simulink model "ClassicalController"  (R2021a)
settings: Solver=VariableStepAuto  StartTime=0.0  StopTime=200  RelTol=1e-3
values from neighbouring files (symbols this model uses):
  Sim_A = m.EquilibriumStateSpace.A    [main.m]
  Sim_B = m.EquilibriumStateSpace.B    [main.m]
  Sim_C = m.EquilibriumStateSpace.C    [main.m]
  Sim_c1_d = sym2poly(d)    [main.m]
  Sim_c1_n = sym2poly(n)    [main.m]
  Sim_c2_d = sym2poly(d)    [main.m]
  Sim_c2_n = sym2poly(n)    [main.m]
settings Model: Creator=james  LastModifiedBy=james

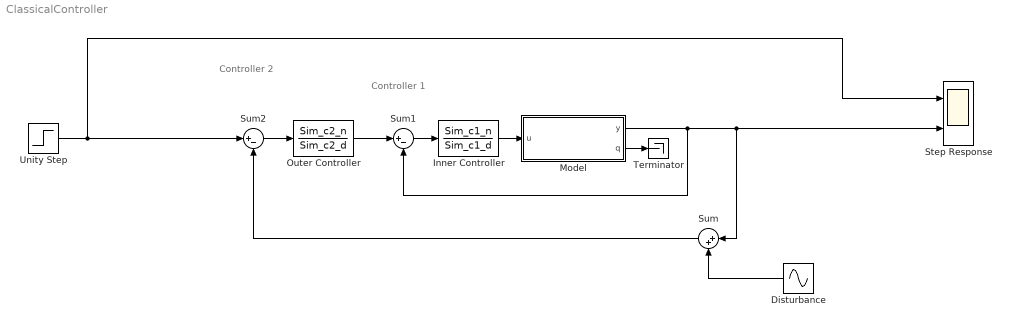
== system ClassicalController ==
  note: Controller 2
  note: Controller 1
  Disturbance : Sin  Amplitude=0.5  Frequency=50  SampleTime=0
  Inner Controller : TransferFcn  Numerator=Sim_c1_n  Denominator=Sim_c1_d
  Model : Subsystem
  Outer Controller : TransferFcn  Numerator=Sim_c2_n  Denominator=Sim_c2_d
  Step Response : Scope  NumInputPorts=2
  Sum : Sum  Inputs=|++
  Sum1 : Sum  Inputs=|+-
  Sum2 : Sum  Inputs=|+-
  Terminator : Terminator
  Unity Step : Step  SampleTime=0
  wires:
  Model/1(y) -> Sum1/2, Sum/1, Step Response/2
  Sum1/1 -> Inner Controller/1
  Model/2(q) -> Terminator/1
  Inner Controller/1 -> Model/1(u)
  Outer Controller/1 -> Sum1/1
  Sum2/1 -> Outer Controller/1
  Unity Step/1 -> Sum2/1, Step Response/1
  Sum/1 -> Sum2/2
  Disturbance/1 -> Sum/2

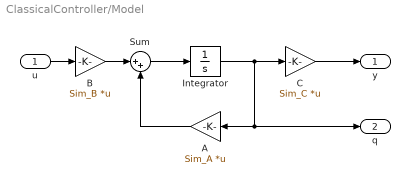
== system ClassicalController/Model ==
  u : Inport
  A : Gain  Gain=Sim_A  Multiplication=Matrix(K*u)
  B : Gain  Gain=Sim_B  Multiplication=Matrix(K*u)
  C : Gain  Gain=Sim_C  Multiplication=Matrix(K*u)
  Integrator : Integrator
  Sum : Sum  Inputs=|++
  y : Outport
  q : Outport  Port=2
  wires:
  B/1 -> Sum/1
  C/1 -> y/1
  Integrator/1 -> q/1, A/1, C/1
  u/1 -> B/1
  Sum/1 -> Integrator/1
  A/1 -> Sum/2
